simulink model "Lab1"  (R2019b)
settings: Solver=ode4  StartTime=0.0  StopTime=SimulationTime  FixedStep=0.01  RelTol=1e-3
values from neighbouring files (symbols this model uses):
  FinalVoltage = 0    [ScriptLab1.m]    (also in Zadanie1.m; Zadanie2.m = values(i); Zadanie3.m = 1; Zadanie4.m)
  InitialVoltage = 3    [ScriptLab1.m]    (also in Zadanie1.m = 0; Zadanie2.m = values(i); Zadanie3.m = 1; Zadanie4.m)
  K = 1/RC(i)    [ScriptLab1.m]    (also in Zadanie1.m = 1 /(R * C); Zadanie4.m = 1/ (Rv(i) * C); Zadanie5.m)
  StepTime = 5    [ScriptLab1.m]    (also in Zadanie1.m = 0; Zadanie2.m = 0; Zadanie3.m = 0; Zadanie4.m)
  WPC = 0    [ScriptLab1.m]    (also in Zadanie1.m = WPCv(i); Zadanie2.m; Zadanie3.m = values(i); Zadanie4.m)
settings Model: Creator=falcon  LastModifiedBy=falcon
settings DataIOCC: LimitDataPoints=on

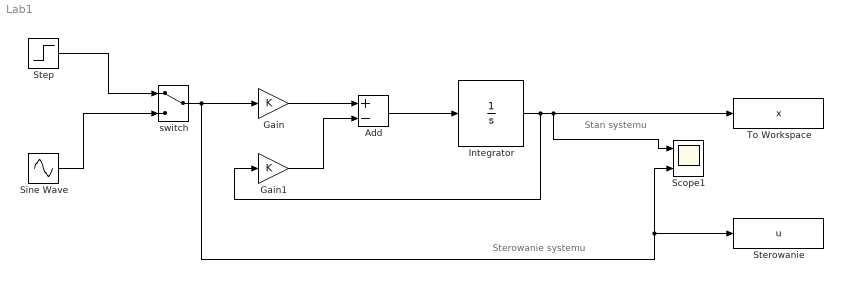
== system Lab1 ==
  note: Sterowanie systemu
  note: Stan systemu
  Add : Sum  Inputs=+-
  Gain : Gain  Gain=K
  Gain1 : Gain  Gain=K
  Integrator : Integrator  InitialCondition=WPC
  Scope1 : Scope  NumInputPorts=2
  Sine Wave : Sin  Frequency=62  SampleTime=0
  Step : Step  Time=StepTime  Before=InitialVoltage  After=FinalVoltage  SampleTime=0
  "Sterowanie " : ToWorkspace  VariableName=u  SampleTime=-1
  To Workspace : ToWorkspace  VariableName=x  SampleTime=-1
  switch : ManualSwitch
  wires:
  Sine Wave/1 -> switch/2
  switch/1 -> Scope1/2, "Sterowanie "/1, Gain/1
  Add/1 -> Integrator/1
  Integrator/1 -> Gain1/1, To Workspace/1, Scope1/1
  Gain/1 -> Add/1
  Gain1/1 -> Add/2
  Step/1 -> switch/1
